simulink model "linmodel_eq2_discr"  (R2019a)
settings: Solver=VariableStepAuto  StartTime=0.0  StopTime=30  RelTol=1e-3
InitFcn:
  | lin_discr_model
undefined symbols (not defined in the file): A_eq2_d, B_eq2_d, C_eq2_d, D_eq2_d, Discrete, Time, Ts
libraries: ctrlSharedLib x1
settings Model: Creator=jessi  LastModifiedBy=jessi

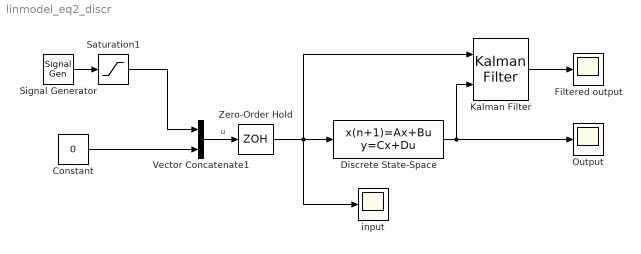
== system linmodel_eq2_discr ==
  Constant : Constant  Value=0
  "Discrete State-Space " : DiscreteStateSpace  A=A_eq2_d  B=B_eq2_d  C=C_eq2_d  D=D_eq2_d  InitialCondition=[0;0;0;0]  SampleTime=Ts
  Filtered output : Scope
  Kalman Filter : ctrlSharedLib/Kalman Filter  TimeDomain=Discrete-Time  UseCurrentEstimator=on  ModelSource=Individual A, B, C, D matrices  ModelSourceVariable=ss(0.95,1,1,0,1)  A=A_eq2_d  B=B_eq2_d  C=C_eq2_d  D=D_eq2_d  NumberOfStates=1  NumberOfInputs=1  NumberOfOutputs=1  InitialEstimateSource=Dialog  X0=[0;0;0;0]  P0=10  UseK=off  UseGH=off  NumberOfProcessNoiseInputs=1  G=1  TimeInvariantG=on  H=0  TimeInvariantH=on  Q=([0,0,0,0])  TimeInvariantQ=on  R=([0.0001,0.0001])  TimeInvariantR=on  N=0  TimeInvariantN=on  AddInputPort=on  AddEnablePort=off  OutputEstimatedY=off  OutputP=off  Ts=-1
      settings: SourceProductBaseCode=CT
  Output : Scope
  Saturation1 : Saturate  UpperLimit=1  LowerLimit=-1
  Signal Generator : SignalGenerator  WaveForm=square  Amplitude=0.3
  Vector Concatenate1 : Concatenate
  Zero-Order Hold : ZeroOrderHold  SampleTime=Ts
  input : Scope
  wires:
  Constant/1 -> Vector Concatenate1/2
  Signal Generator/1 -> Saturation1/1
  Saturation1/1 -> Vector Concatenate1/1
  Vector Concatenate1/1 -> Zero-Order Hold/1  "u"
  Zero-Order Hold/1 -> input/1, Kalman Filter/1, "Discrete State-Space "/1
  "Discrete State-Space "/1 -> Kalman Filter/2, Output/1
  Kalman Filter/1 -> Filtered output/1
